simulink model "fullVehicleModel_17b"  (R2017b)
settings: Solver=VariableStepAuto  StartTime=0.0  StopTime=10.0  RelTol=1e-3
undefined symbols (not defined in the file): ambient_temp, bat, bat_r1, Batt, batt_initCharge, Batt_sensorLag_s, bvatt_AhRating, DiscIntNeverNeededParam, electronics_power, env, module_broad_area, module_small_area, module_top_area, mot, no_module, shifterPos, Ts, Ts_elec
libraries: Soft_ECUs x90, fl_lib x67, nesl_utility x29, Battery_lib x28, Gen_lib x13, simulink x10, aerolibconvert2 x7, SoftCAN_Interface x6, autolibshared x2, Additional_blocks_lib x1, elec_lib x1
(part 3 of 4)

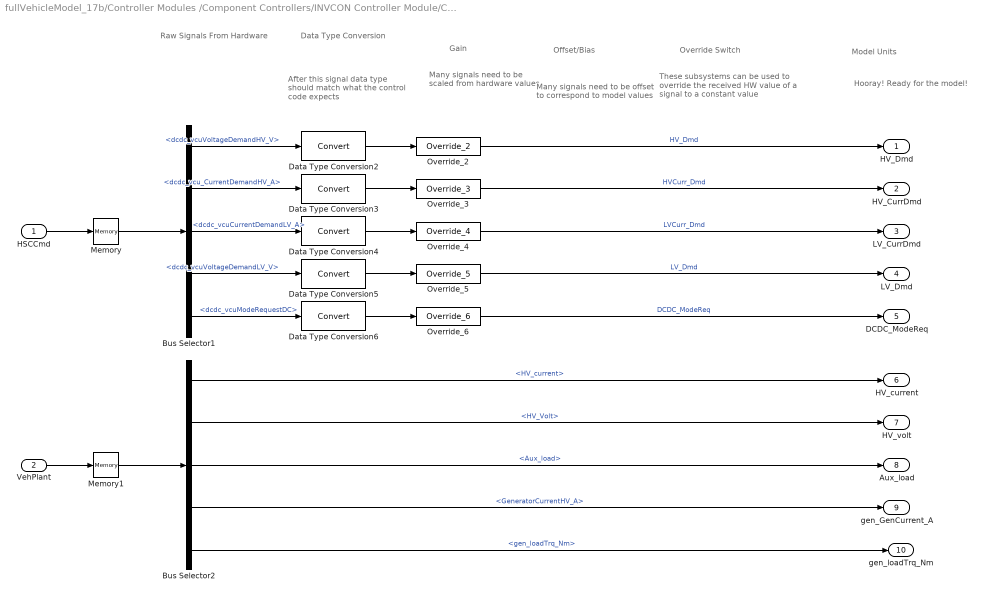
== system fullVehicleModel_17b/Controller Modules /Component Controllers/INVCON Controller Module/Controller Inputs/SiL Inputs ==
  note: Override Switch
  note: These subsystems can be used
      |  to override the received HW value
      | of a signal to a constant value
  note: Offset/Bias
  note: Many signals need
      | to be scaled from
      | hardware values
  note: Gain
  note: Raw Signals
      | From Hardware
  note: Model Units
  note: Hooray! Ready for
      | the model!
  note: After this signal data
      | type should match what
      | the control code expects
  note: Data Type
      | Conversion
  note: Many signals need
      | to be offset to correspond
      | to model values
  HSCCmd : Inport
  VehPlant : Inport  Port=2
  Bus Selector1 : BusSelector  OutputSignals=dcdc_vcuVoltageDemandHV_V,dcdc_vcu_CurrentDemandHV_A,dcdc_vcuCurrentDemandLV_A,dcdc_vcuVoltageDemandLV_V,dcdc_vcuModeRequestDC
  Bus Selector2 : BusSelector  OutputSignals=HV_current,HV_Volt,Aux_load,GeneratorCurrentHV_A,gen_loadTrq_Nm
  Data Type Conversion{2..6} (5 alike) : DataTypeConversion
  Memory : Memory
  Memory1 : Memory
  Override_2 : Gen_lib/INVCON_SoftECU2/SignalIn_Conversion_FIU/Override_2
  Override_3 : Gen_lib/INVCON_SoftECU2/SignalIn_Conversion_FIU/Override_3
  Override_4 : Gen_lib/INVCON_SoftECU2/SignalIn_Conversion_FIU/Override_4
  Override_5 : Gen_lib/INVCON_SoftECU2/SignalIn_Conversion_FIU/Override_5
  Override_6 : Gen_lib/INVCON_SoftECU2/SignalIn_Conversion_FIU/Override_6
  HV_Dmd : Outport
  HV_CurrDmd : Outport  Port=2
  LV_CurrDmd : Outport  Port=3
  LV_Dmd : Outport  Port=4
  DCDC_ModeReq : Outport  Port=5
  HV_current : Outport  Port=6
  HV_volt : Outport  Port=7
  Aux_load : Outport  Port=8
  gen_GenCurrent_A : Outport  Port=9
  gen_loadTrq_Nm : Outport  Port=10
  wires:
  Bus Selector1/4 -> Data Type Conversion5/1  "<dcdc_vcuVoltageDemandLV_V>"
  Override_6/1 -> DCDC_ModeReq/1  "DCDC_ModeReq"
  Override_3/1 -> HV_CurrDmd/1  "HVCurr_Dmd"
  Override_4/1 -> LV_CurrDmd/1  "LVCurr_Dmd"
  Bus Selector1/2 -> Data Type Conversion3/1  "<dcdc_vcu_CurrentDemandHV_A>"
  Bus Selector1/5 -> Data Type Conversion6/1  "<dcdc_vcuModeRequestDC>"
  Override_2/1 -> HV_Dmd/1  "HV_Dmd"
  Data Type Conversion5/1 -> Override_5/1
  Bus Selector1/3 -> Data Type Conversion4/1  "<dcdc_vcuCurrentDemandLV_A>"
  Data Type Conversion3/1 -> Override_3/1
  HSCCmd/1 -> Memory/1
  Data Type Conversion6/1 -> Override_6/1
  Bus Selector1/1 -> Data Type Conversion2/1  "<dcdc_vcuVoltageDemandHV_V>"
  Data Type Conversion2/1 -> Override_2/1
  Override_5/1 -> LV_Dmd/1  "LV_Dmd"
  Data Type Conversion4/1 -> Override_4/1
  Memory/1 -> Bus Selector1/1
  Bus Selector2/5 -> gen_loadTrq_Nm/1  "<gen_loadTrq_Nm>"
  Bus Selector2/2 -> HV_volt/1  "<HV_Volt>"
  Bus Selector2/1 -> HV_current/1  "<HV_current>"
  Bus Selector2/4 -> gen_GenCurrent_A/1  "<GeneratorCurrentHV_A>"
  Bus Selector2/3 -> Aux_load/1  "<Aux_load>"
  Memory1/1 -> Bus Selector2/1
  VehPlant/1 -> Memory1/1

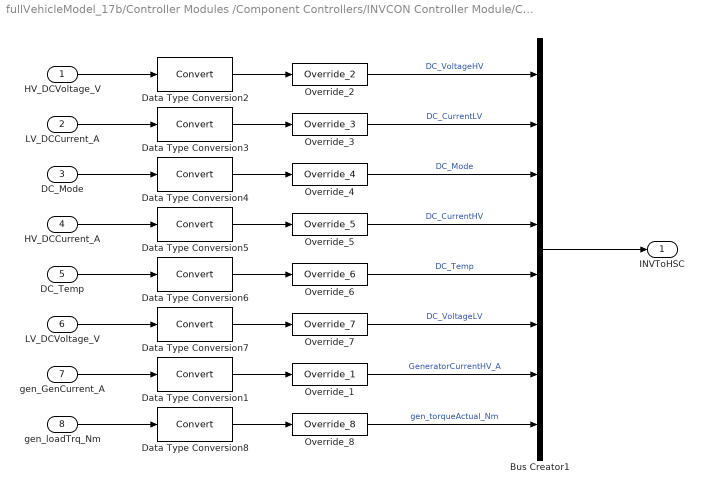
== system fullVehicleModel_17b/Controller Modules /Component Controllers/INVCON Controller Module/Controller Outputs/SiL Controller Outputs ==
  HV_DCVoltage_V : Inport
  LV_DCCurrent_A : Inport  Port=2
  DC_Mode : Inport  Port=3
  HV_DCCurrent_A : Inport  Port=4
  DC_Temp : Inport  Port=5
  LV_DCVoltage_V : Inport  Port=6
  gen_GenCurrent_A : Inport  Port=7
  gen_loadTrq_Nm : Inport  Port=8
  Bus Creator1 : BusCreator  Inputs=8
  Data Type Conversion{1..8} (8 alike) : DataTypeConversion
  Override_1 : Gen_lib/INVCON_SoftECU2/SignalOut_Conversion_FIU/Override_1
  Override_2 : Gen_lib/INVCON_SoftECU2/SignalOut_Conversion_FIU/Override_2
  Override_3 : Gen_lib/INVCON_SoftECU2/SignalOut_Conversion_FIU/Override_3
  Override_4 : Gen_lib/INVCON_SoftECU2/SignalOut_Conversion_FIU/Override_4
  Override_5 : Gen_lib/INVCON_SoftECU2/SignalOut_Conversion_FIU/Override_5
  Override_6 : Gen_lib/INVCON_SoftECU2/SignalOut_Conversion_FIU/Override_6
  Override_7 : Gen_lib/INVCON_SoftECU2/SignalOut_Conversion_FIU/Override_7
  Override_8 : Gen_lib/INVCON_SoftECU2/SignalOut_Conversion_FIU/Override_8
  INVToHSC : Outport
  wires:
  Data Type Conversion8/1 -> Override_8/1
  Data Type Conversion3/1 -> Override_3/1
  Override_8/1 -> Bus Creator1/8  "gen_torqueActual_Nm"
  Bus Creator1/1 -> INVToHSC/1
  Data Type Conversion4/1 -> Override_4/1
  Data Type Conversion2/1 -> Override_2/1
  Override_2/1 -> Bus Creator1/1  "DC_VoltageHV"
  Override_1/1 -> Bus Creator1/7  "GeneratorCurrentHV_A"
  Data Type Conversion5/1 -> Override_5/1
  Data Type Conversion6/1 -> Override_6/1
  Data Type Conversion7/1 -> Override_7/1
  Data Type Conversion1/1 -> Override_1/1
  Override_4/1 -> Bus Creator1/3  "DC_Mode"
  Override_7/1 -> Bus Creator1/6  "DC_VoltageLV"
  Override_3/1 -> Bus Creator1/2  "DC_CurrentLV"
  Override_6/1 -> Bus Creator1/5  "DC_Temp"
  Override_5/1 -> Bus Creator1/4  "DC_CurrentHV"
  HV_DCVoltage_V/1 -> Data Type Conversion2/1
  LV_DCCurrent_A/1 -> Data Type Conversion3/1
  DC_Mode/1 -> Data Type Conversion4/1
  HV_DCCurrent_A/1 -> Data Type Conversion5/1
  DC_Temp/1 -> Data Type Conversion6/1
  LV_DCVoltage_V/1 -> Data Type Conversion7/1
  gen_GenCurrent_A/1 -> Data Type Conversion1/1
  gen_loadTrq_Nm/1 -> Data Type Conversion8/1

== system fullVehicleModel_17b/Controller Modules /Component Controllers/INVCON Controller Module/INVCON Controller Module/Conditional Divide ==
  u1 : Inport
  u2 : Inport  Port=2
  u3 : Inport  Port=3
  Constant1 : Constant  Value=eps
  Constant3 : Constant  Value=0
  Divide : Product  Inputs=/*
  Logical Operator : Logic  Operator=NOT  AllPortsSameDT=off  OutDataTypeStr=boolean
  Relational Operator : RelationalOperator  Operator===  OutDataTypeStr=boolean  RndMeth=Nearest
  Switch : Switch  Criteria=u2 ~= 0
  Switch1 : Switch  Criteria=u2 ~= 0
  Out1 : Outport
  wires:
  Constant3/1 -> Relational Operator/2
  Divide/1 -> Switch1/1
  u2/1 -> Relational Operator/1, Switch/3
  u1/1 -> Divide/2
  Relational Operator/1 -> Switch/2, Logical Operator/1
  u3/1 -> Switch1/3
  Constant1/1 -> Switch/1
  Switch1/1 -> Out1/1
  Logical Operator/1 -> Switch1/2
  Switch/1 -> Divide/1

== system fullVehicleModel_17b/Controller Modules /Component Controllers/Left Motor Control Module/Controller/Fault Daignosis ==
  current : Inport
  voltage : Inport  Port=2
  temp : Inport  Port=3
  Bus Creator : BusCreator  Inputs=5
  Device Temp to High : Subsystem
  Motor Temp to High : Subsystem
  No Power Supply Voltage : Subsystem
  Over Current : Subsystem
  Over Voltage : Subsystem
  Fault Message : Outport
  wires:
  Bus Creator/1 -> Fault Message/1
  Over Current/1(Out1) -> Bus Creator/5  "mot_fault_iPeak"
  Over Voltage/1(Out1) -> Bus Creator/2  "mot_fault_overVoltage"
  Device Temp to High/1(Out1) -> Bus Creator/4  "mot_fault_deviceTemp"
  Motor Temp to High/1(Out1) -> Bus Creator/3  "mot_fault_mtrTemp"
  No Power Supply Voltage/1(Out1) -> Bus Creator/1  "mot_fault_pwrVoltage"
  temp/1 -> Motor Temp to High/1(Mot_temp), Device Temp to High/1(Device Temp)
  current/1 -> Over Current/1(Motor Current)
  voltage/1 -> Over Voltage/1(Device Voltage), No Power Supply Voltage/1(mot_voltage)

== system fullVehicleModel_17b/Controller Modules /Component Controllers/Left Motor Control Module/Controller/Motor CMD ==
  note: This subsystem is used to override the model value of a signal to a constant value
  note: Override Switch Subsystem
  trq_cmd : Inport
  mot_mode : Inport  Port=2
  Multiport Switch : MultiPortSwitch  DataPortOrder=Zero-based contiguous  Inputs=2  zeroidx=on
  Override Value : Constant  Value=0
  Out1 : Outport
  wires:
  mot_mode/1 -> Multiport Switch/1
  Override Value/1 -> Multiport Switch/2
  trq_cmd/1 -> Multiport Switch/3
  Multiport Switch/1 -> Out1/1

== system fullVehicleModel_17b/Controller Modules /Component Controllers/Left Motor Control Module/Controller/Subsystem ==
  voltage : Inport
  speed : Inport  Port=2
  current : Inport  Port=3
  mode : Inport  Port=4
  Out1 : Outport

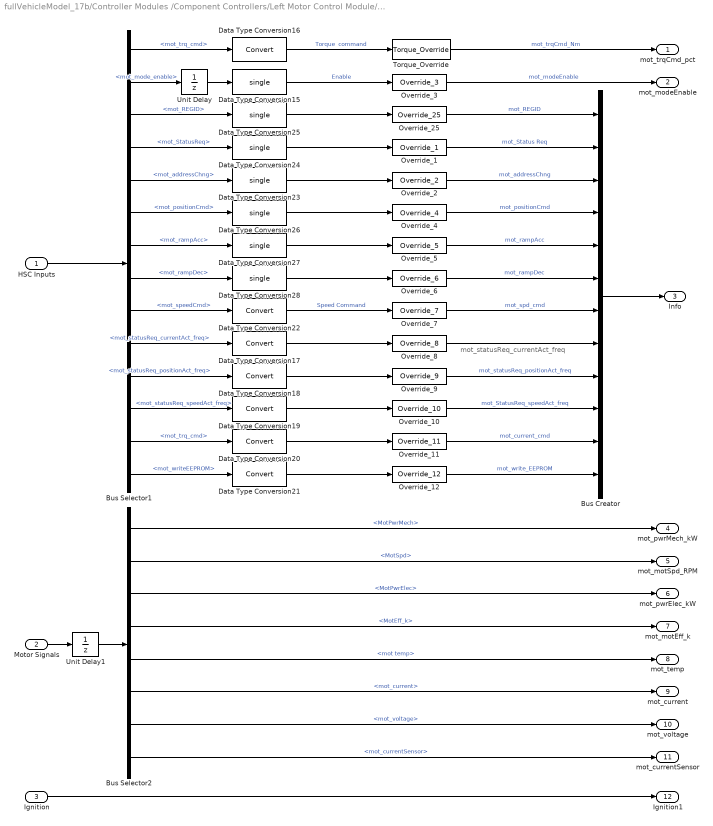
== system fullVehicleModel_17b/Controller Modules /Component Controllers/Left Motor Control Module/Controller Inputs/SiL Inputs ==
  note: mot_statusReq_currentAct_freq
  HSC Inputs : Inport
  Motor Signals : Inport  Port=2
  Ignition : Inport  Port=3
  Bus Creator : BusCreator  Inputs=12
  Bus Selector1 : BusSelector  OutputSignals=mot_trq_cmd,mot_mode_enable,mot_REGID,mot_StatusReq,mot_addressChng,mot_positionCmd,mot_rampAcc,mot_rampDec,mot_speedCmd,mot_statusReq_currentAct_freq,mot_statusReq_positionAct_freq,mot_statusReq_speedAct_freq,mot_trq_cmd,mot_writeEEPROM
  Bus Selector2 : BusSelector  OutputSignals=MotPwrMech,MotSpd,MotPwrElec,MotEff_k,mot temp,mot_current,mot_voltage,mot_currentSensor
  Data Type Conversion{15,23..28} (7 alike) : DataTypeConversion  OutDataTypeStr=single
  Data Type Conversion{16..22} (7 alike) : DataTypeConversion
  Override_1 : Soft_ECUs/softECU_Motor/Conversion/Override_1
  Override_10 : Soft_ECUs/softECU_Motor/Conversion/Override_10
  Override_11 : Soft_ECUs/softECU_Motor/Conversion/Override_11
  Override_12 : Soft_ECUs/softECU_Motor/Conversion/Override_12
  Override_2 : Soft_ECUs/softECU_Motor/Conversion/Override_2
  Override_25 : Soft_ECUs/softECU_Motor/Conversion/Override_25
  Override_3 : Soft_ECUs/softECU_Motor/Conversion/Override_3
  Override_4 : Soft_ECUs/softECU_Motor/Conversion/Override_4
  Override_5 : Soft_ECUs/softECU_Motor/Conversion/Override_5
  Override_6 : Soft_ECUs/softECU_Motor/Conversion/Override_6
  Override_7 : Soft_ECUs/softECU_Motor/Conversion/Override_7
  Override_8 : Soft_ECUs/softECU_Motor/Conversion/Override_8
  Override_9 : Soft_ECUs/softECU_Motor/Conversion/Override_9
  Torque_Override : Soft_ECUs/softECU_Motor/Conversion/Torque_Override
  Unit Delay : UnitDelay  SampleTime=-1
  Unit Delay1 : UnitDelay  SampleTime=-1
  mot_trqCmd_pct : Outport
  mot_modeEnable : Outport  Port=2
  Info : Outport  Port=3
  mot_pwrMech_kW : Outport  Port=4
  mot_motSpd_RPM : Outport  Port=5
  mot_pwrElec_kW : Outport  Port=6
  mot_motEff_k : Outport  Port=7
  mot_temp : Outport  Port=8
  mot_current : Outport  Port=9
  mot_voltage : Outport  Port=10
  mot_currentSensor : Outport  Port=11
  Ignition1 : Outport  Port=12
  wires:
  Override_12/1 -> Bus Creator/12  "mot_write_EEPROM"
  Data Type Conversion24/1 -> Override_1/1
  Bus Selector1/14 -> Data Type Conversion21/1  "<mot_writeEEPROM>"
  Override_6/1 -> Bus Creator/6  "mot_rampDec"
  Bus Selector1/13 -> Data Type Conversion20/1  "<mot_trq_cmd>"
  Override_1/1 -> Bus Creator/2  "mot_Status Req"
  Bus Selector1/7 -> Data Type Conversion27/1  "<mot_rampAcc>"
  Data Type Conversion22/1 -> Override_7/1  "Speed Command"
  Bus Selector1/12 -> Data Type Conversion19/1  "<mot_statusReq_speedAct_freq>"
  Data Type Conversion17/1 -> Override_8/1
  Data Type Conversion18/1 -> Override_9/1
  Override_9/1 -> Bus Creator/9  "mot_statusReq_positionAct_freq"
  Bus Selector1/11 -> Data Type Conversion18/1  "<mot_statusReq_positionAct_freq>"
  Override_10/1 -> Bus Creator/10  "mot_StatusReq_speedAct_freq"
  Override_4/1 -> Bus Creator/4  "mot_positionCmd"
  Data Type Conversion27/1 -> Override_5/1
  Override_8/1 -> Bus Creator/8
  Data Type Conversion23/1 -> Override_2/1
  Override_11/1 -> Bus Creator/11  "mot_current_cmd"
  Data Type Conversion25/1 -> Override_25/1
  Bus Selector1/6 -> Data Type Conversion26/1  "<mot_positionCmd>"
  Data Type Conversion28/1 -> Override_6/1
  Override_7/1 -> Bus Creator/7  "mot_spd_cmd"
  Bus Selector1/5 -> Data Type Conversion23/1  "<mot_addressChng>"
  Data Type Conversion26/1 -> Override_4/1
  Bus Selector1/8 -> Data Type Conversion28/1  "<mot_rampDec>"
  Bus Selector1/1 -> Data Type Conversion16/1  "<mot_trq_cmd>"
  Data Type Conversion19/1 -> Override_10/1
  Bus Selector1/3 -> Data Type Conversion25/1  "<mot_REGID>"
  Override_25/1 -> Bus Creator/1  "mot_REGID"
  Bus Selector1/4 -> Data Type Conversion24/1  "<mot_StatusReq>"
  Data Type Conversion21/1 -> Override_12/1
  Override_2/1 -> Bus Creator/3  "mot_addressChng"
  Data Type Conversion16/1 -> Torque_Override/1  "Torque  command"
  Override_5/1 -> Bus Creator/5  "mot_rampAcc"
  Bus Selector1/2 -> Unit Delay/1  "<mot_mode_enable>"
  Bus Selector1/9 -> Data Type Conversion22/1  "<mot_speedCmd>"
  Unit Delay/1 -> Data Type Conversion15/1
  HSC Inputs/1 -> Bus Selector1/1
  Data Type Conversion15/1 -> Override_3/1  "Enable"
  Bus Selector1/10 -> Data Type Conversion17/1  "<mot_statusReq_currentAct_freq>"
  Data Type Conversion20/1 -> Override_11/1
  Bus Selector2/5 -> mot_temp/1  "<mot temp>"
  Bus Selector2/6 -> mot_current/1  "<mot_current>"
  Bus Selector2/4 -> mot_motEff_k/1  "<MotEff_k>"
  Bus Selector2/3 -> mot_pwrElec_kW/1  "<MotPwrElec>"
  Bus Selector2/2 -> mot_motSpd_RPM/1  "<MotSpd>"
  Bus Selector2/1 -> mot_pwrMech_kW/1  "<MotPwrMech>"
  Motor Signals/1 -> Unit Delay1/1
  Bus Selector2/7 -> mot_voltage/1  "<mot_voltage>"
  Bus Selector2/8 -> mot_currentSensor/1  "<mot_currentSensor>"
  Bus Creator/1 -> Info/1
  Override_3/1 -> mot_modeEnable/1  "mot_modeEnable"
  Torque_Override/1 -> mot_trqCmd_pct/1  "mot_trqCmd_Nm"
  Ignition/1 -> Ignition1/1
  Unit Delay1/1 -> Bus Selector2/1

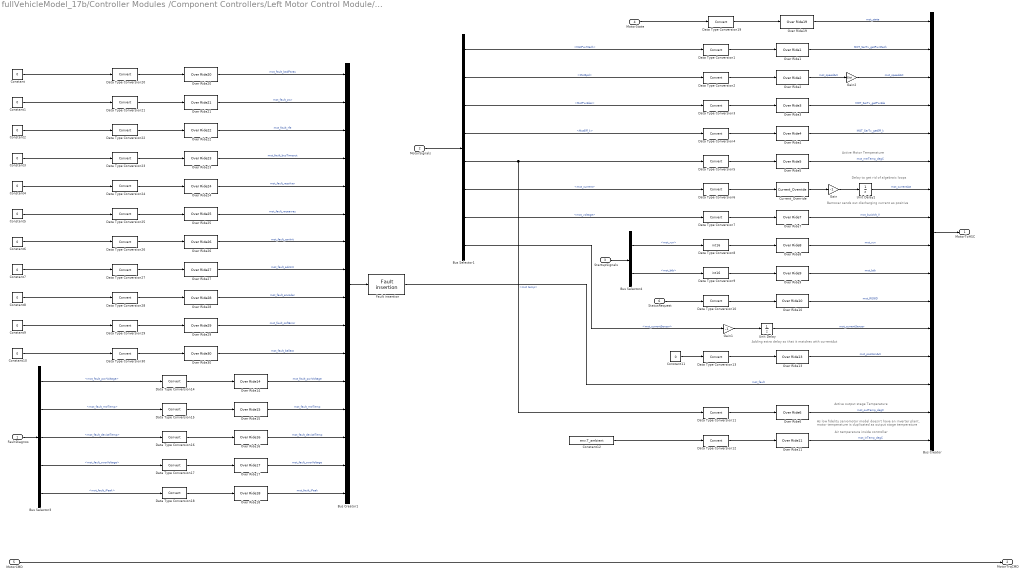
== system fullVehicleModel_17b/Controller Modules /Component Controllers/Left Motor Control Module/Controller Outputs/SiL Controller Outputs ==
  note: Active Motor Temperature
  note: Adding extra delay so that it matches with currentAct
  note: As low fidelity servomotor model doesn't have an inverter plant,
      | motor temperature is duplicated as output stage temperature
  note: Air temperature inside controller
  note: Delay to get rid of algebraic loops
  note: Active output stage Temperature
  note: Bamocar sends out discharging current as positive
  FaultDiagnos : Inport
  MotorSignals : Inport  Port=2
  StartupSignals : Inport  Port=3
  MotorState : Inport  Port=4
  MotorCMD : Inport  Port=5
  StatusRequest : Inport  Port=6
  Bus Creator : BusCreator  Inputs=16
  Bus Creator1 : BusCreator  Inputs=16
  Bus Selector1 : BusSelector  OutputSignals=MotPwrMech,MotSpd,MotPwrElec,MotEff_k,mot temp,mot_current,mot_voltage,mot_currentSensor
  Bus Selector3 : BusSelector  OutputSignals=mot_fault_pwrVoltage,mot_fault_mtrTemp,mot_fault_deviceTemp,mot_fault_overVoltage,mot_fault_iPeak
  Bus Selector4 : BusSelector  OutputSignals=mot_run,mot_btb
  Constant{,1..11} (12 alike) : Constant  Value=0
  Constant12 : Constant  Value=env.T_ambient
  Current_Override : Soft_ECUs/softECU_Motor/conversion 2/Current_Override
  Data Type Conversion{1..7,10..30} (28 alike) : DataTypeConversion
  Data Type Conversion8 : DataTypeConversion  OutDataTypeStr=int16
  Data Type Conversion9 : DataTypeConversion  OutDataTypeStr=int16
  Fault insertion : Soft_ECUs/softECU_Motor/conversion 2/Fault insertion
  Gain : Gain  Gain=-1
  Gain1 : Gain  Gain=-1
  Gain2 : Gain  Gain=30/pi
  Over Ride1 : Soft_ECUs/softECU_Motor/conversion 2/Over Ride1
  Over Ride10 : Soft_ECUs/softECU_Motor/conversion 2/Over Ride10
  Over Ride11 : Soft_ECUs/softECU_Motor/conversion 2/Over Ride11
  Over Ride13 : Soft_ECUs/softECU_Motor/conversion 2/Over Ride13
  Over Ride14 : Soft_ECUs/softECU_Motor/conversion 2/Over Ride14
  Over Ride15 : Soft_ECUs/softECU_Motor/conversion 2/Over Ride15
  Over Ride16 : Soft_ECUs/softECU_Motor/conversion 2/Over Ride16
  Over Ride17 : Soft_ECUs/softECU_Motor/conversion 2/Over Ride17
  Over Ride18 : Soft_ECUs/softECU_Motor/conversion 2/Over Ride18
  Over Ride19 : Soft_ECUs/softECU_Motor/conversion 2/Over Ride19
  Over Ride2 : Soft_ECUs/softECU_Motor/conversion 2/Over Ride2
  Over Ride20 : Soft_ECUs/softECU_Motor/conversion 2/Over Ride20
  Over Ride21 : Soft_ECUs/softECU_Motor/conversion 2/Over Ride21
  Over Ride22 : Soft_ECUs/softECU_Motor/conversion 2/Over Ride22
  Over Ride23 : Soft_ECUs/softECU_Motor/conversion 2/Over Ride23
  Over Ride24 : Soft_ECUs/softECU_Motor/conversion 2/Over Ride24
  Over Ride25 : Soft_ECUs/softECU_Motor/conversion 2/Over Ride25
  Over Ride26 : Soft_ECUs/softECU_Motor/conversion 2/Over Ride26
  Over Ride27 : Soft_ECUs/softECU_Motor/conversion 2/Over Ride27
  Over Ride28 : Soft_ECUs/softECU_Motor/conversion 2/Over Ride28
  Over Ride29 : Soft_ECUs/softECU_Motor/conversion 2/Over Ride29
  Over Ride3 : Soft_ECUs/softECU_Motor/conversion 2/Over Ride3
  Over Ride30 : Soft_ECUs/softECU_Motor/conversion 2/Over Ride30
  Over Ride4 : Soft_ECUs/softECU_Motor/conversion 2/Over Ride4
  Over Ride5 : Soft_ECUs/softECU_Motor/conversion 2/Over Ride5
  Over Ride6 : Soft_ECUs/softECU_Motor/conversion 2/Over Ride6
  Over Ride7 : Soft_ECUs/softECU_Motor/conversion 2/Over Ride7
  Over Ride8 : Soft_ECUs/softECU_Motor/conversion 2/Over Ride8
  Over Ride9 : Soft_ECUs/softECU_Motor/conversion 2/Over Ride9
  Unit Delay : UnitDelay  SampleTime=-1
  Unit Delay1 : UnitDelay  SampleTime=-1
  MotorToHSC : Outport
  MotorTrqCMD : Outport  Port=2
  wires:
  Data Type Conversion13/1 -> Over Ride13/1
  Over Ride10/1 -> Bus Creator/11  "mot_REGID"
  StatusRequest/1 -> Data Type Conversion10/1
  MotorState/1 -> Data Type Conversion19/1
  Over Ride8/1 -> Bus Creator/9  "mot_run"
  Constant10/1 -> Data Type Conversion30/1
  Bus Selector1/3 -> Data Type Conversion3/1  "<MotPwrElec>"
  Over Ride9/1 -> Bus Creator/10  "mot_btb"
  Data Type Conversion9/1 -> Over Ride9/1
  Data Type Conversion21/1 -> Over Ride21/1
  StartupSignals/1 -> Bus Selector4/1
  MotorSignals/1 -> Bus Selector1/1
  Bus Selector4/2 -> Data Type Conversion9/1  "<mot_btb>"
  Bus Selector1/2 -> Data Type Conversion2/1  "<MotSpd>"
  Data Type Conversion5/1 -> Over Ride5/1
  Data Type Conversion28/1 -> Over Ride28/1
  Bus Selector4/1 -> Data Type Conversion8/1  "<mot_run>"
  Bus Selector1/7 -> Data Type Conversion7/1  "<mot_voltage>"
  Current_Override/1 -> Gain/1
  Bus Selector3/1 -> Data Type Conversion14/1  "<mot_fault_pwrVoltage>"
  Over Ride18/1 -> Bus Creator1/16  "mot_fault_iPeak"
  Over Ride16/1 -> Bus Creator1/14  "mot_fault_deviceTemp"
  Over Ride14/1 -> Bus Creator1/12  "mot_fault_pwrVoltage"
  Data Type Conversion1/1 -> Over Ride1/1
  Constant9/1 -> Data Type Conversion29/1
  Constant/1 -> Data Type Conversion20/1
  Data Type Conversion10/1 -> Over Ride10/1
  Data Type Conversion23/1 -> Over Ride23/1
  Data Type Conversion3/1 -> Over Ride3/1
  Data Type Conversion8/1 -> Over Ride8/1
  Data Type Conversion4/1 -> Over Ride4/1
  Bus Selector1/1 -> Data Type Conversion1/1  "<MotPwrMech>"
  Bus Selector1/5 -> Data Type Conversion5/1, Data Type Conversion11/1  "<mot temp>"
  Over Ride3/1 -> Bus Creator/4  "MOT_SerTx_getPwrEle"
  Over Ride5/1 -> Bus Creator/6  "mot_mtrTemp_degC"
  FaultDiagnos/1 -> Bus Selector3/1
  Bus Selector3/2 -> Data Type Conversion15/1  "<mot_fault_mtrTemp>"
  Bus Selector3/3 -> Data Type Conversion16/1  "<mot_fault_deviceTemp>"
  Data Type Conversion20/1 -> Over Ride20/1
  Constant11/1 -> Data Type Conversion13/1
  Data Type Conversion24/1 -> Over Ride24/1
  Over Ride7/1 -> Bus Creator/8  "mot_busVolt_V"
  Data Type Conversion19/1 -> Over Ride19/1
  Over Ride13/1 -> Bus Creator/13  "mot_positionAct"
  Over Ride19/1 -> Bus Creator/1  "mot_state"
  Bus Creator1/1 -> Fault insertion/1
  Data Type Conversion22/1 -> Over Ride22/1
  Gain2/1 -> Bus Creator/3  "mot_speedAct"
  Over Ride21/1 -> Bus Creator1/2  "mot_fault_pwr"
  Over Ride15/1 -> Bus Creator1/13  "mot_fault_mtrTemp"
  Data Type Conversion2/1 -> Over Ride2/1
  Data Type Conversion7/1 -> Over Ride7/1
  Over Ride20/1 -> Bus Creator1/1  "mot_fault_badParas"
  Data Type Conversion30/1 -> Over Ride30/1
  Bus Creator/1 -> MotorToHSC/1
  Over Ride6/1 -> Bus Creator/15  "mot_outTemp_degC"
  Over Ride25/1 -> Bus Creator1/6  "mot_fault_raceaway"
  Bus Selector3/4 -> Data Type Conversion17/1  "<mot_fault_overVoltage>"
  Over Ride1/1 -> Bus Creator/2  "MOT_SerTx_getPwrMech"
  Over Ride30/1 -> Bus Creator1/11  "mot_fault_ballast"
  Constant7/1 -> Data Type Conversion27/1
  Unit Delay/1 -> Bus Creator/12  "mot_currentSensor"
  Data Type Conversion18/1 -> Over Ride18/1
  Bus Selector1/8 -> Gain1/1  "<mot_currentSensor>"
  Gain1/1 -> Unit Delay/1
  Data Type Conversion11/1 -> Over Ride6/1
  Data Type Conversion12/1 -> Over Ride11/1
  Constant8/1 -> Data Type Conversion28/1
  Data Type Conversion6/1 -> Current_Override/1
  Data Type Conversion16/1 -> Over Ride16/1
  Over Ride22/1 -> Bus Creator1/3  "mot_fault_rfe"
  Constant1/1 -> Data Type Conversion21/1
  Data Type Conversion29/1 -> Over Ride29/1
  Fault insertion/1 -> Bus Creator/14  "mot_fault"
  Constant3/1 -> Data Type Conversion23/1
  Over Ride26/1 -> Bus Creator1/7  "mot_fault_canInit"
  Over Ride4/1 -> Bus Creator/5  "MOT_SerTx_getEff_k"
  Constant2/1 -> Data Type Conversion22/1
  Data Type Conversion14/1 -> Over Ride14/1
  Bus Selector1/4 -> Data Type Conversion4/1  "<MotEff_k>"
  Over Ride11/1 -> Bus Creator/16  "mot_inTemp_degC"
  Data Type Conversion25/1 -> Over Ride25/1
  Constant5/1 -> Data Type Conversion25/1
  Bus Selector1/6 -> Data Type Conversion6/1  "<mot_current>"
  Data Type Conversion26/1 -> Over Ride26/1
  Data Type Conversion27/1 -> Over Ride27/1
  Over Ride24/1 -> Bus Creator1/5  "mot_fault_resolver"
  Gain/1 -> Unit Delay1/1
  Over Ride2/1 -> Gain2/1  "mot_speedAct"
  Unit Delay1/1 -> Bus Creator/7  "mot_currentAct"
  Bus Selector3/5 -> Data Type Conversion18/1  "<mot_fault_iPeak>"
  Over Ride28/1 -> Bus Creator1/9  "mot_fault_encoder"
  Data Type Conversion17/1 -> Over Ride17/1
  Constant12/1 -> Data Type Conversion12/1
  Over Ride27/1 -> Bus Creator1/8  "mot_fault_adcInit"
  Over Ride17/1 -> Bus Creator1/15  "mot_fault_overVoltage"
  Over Ride23/1 -> Bus Creator1/4  "mot_fault_busTimeout"
  Data Type Conversion15/1 -> Over Ride15/1
  Constant6/1 -> Data Type Conversion26/1
  Constant4/1 -> Data Type Conversion24/1
  Over Ride29/1 -> Bus Creator1/10  "mot_fault_softError"
  MotorCMD/1 -> MotorTrqCMD/1

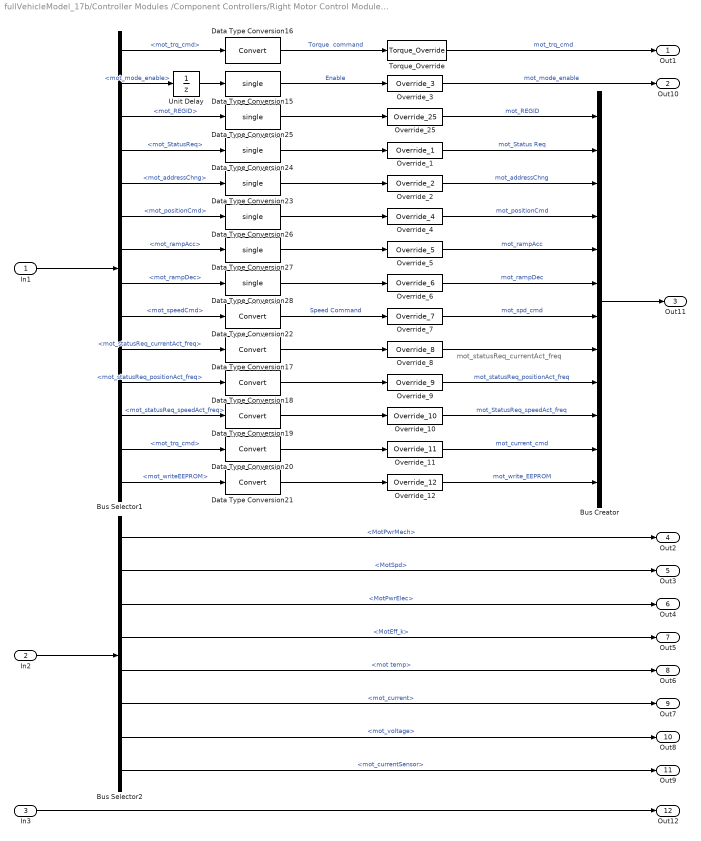
== system fullVehicleModel_17b/Controller Modules /Component Controllers/Right Motor Control Module/Controller Inputs/SiL Inputs ==
  note: mot_statusReq_currentAct_freq
  In1 : Inport
  In2 : Inport  Port=2
  In3 : Inport  Port=3
  Bus Creator : BusCreator  Inputs=12
  Bus Selector1 : BusSelector  OutputSignals=mot_trq_cmd,mot_mode_enable,mot_REGID,mot_StatusReq,mot_addressChng,mot_positionCmd,mot_rampAcc,mot_rampDec,mot_speedCmd,mot_statusReq_currentAct_freq,mot_statusReq_positionAct_freq,mot_statusReq_speedAct_freq,mot_trq_cmd,mot_writeEEPROM
  Bus Selector2 : BusSelector  OutputSignals=MotPwrMech,MotSpd,MotPwrElec,MotEff_k,mot temp,mot_current,mot_voltage,mot_currentSensor
  Data Type Conversion{15,23..28} (7 alike) : DataTypeConversion  OutDataTypeStr=single
  Data Type Conversion{16..22} (7 alike) : DataTypeConversion
  Override_1 : Soft_ECUs/softECU_Motor/Conversion/Override_1
  Override_10 : Soft_ECUs/softECU_Motor/Conversion/Override_10
  Override_11 : Soft_ECUs/softECU_Motor/Conversion/Override_11
  Override_12 : Soft_ECUs/softECU_Motor/Conversion/Override_12
  Override_2 : Soft_ECUs/softECU_Motor/Conversion/Override_2
  Override_25 : Soft_ECUs/softECU_Motor/Conversion/Override_25
  Override_3 : Soft_ECUs/softECU_Motor/Conversion/Override_3
  Override_4 : Soft_ECUs/softECU_Motor/Conversion/Override_4
  Override_5 : Soft_ECUs/softECU_Motor/Conversion/Override_5
  Override_6 : Soft_ECUs/softECU_Motor/Conversion/Override_6
  Override_7 : Soft_ECUs/softECU_Motor/Conversion/Override_7
  Override_8 : Soft_ECUs/softECU_Motor/Conversion/Override_8
  Override_9 : Soft_ECUs/softECU_Motor/Conversion/Override_9
  Torque_Override : Soft_ECUs/softECU_Motor/Conversion/Torque_Override
  Unit Delay : UnitDelay  SampleTime=-1
  Out1 : Outport
  Out10 : Outport  Port=2
  Out11 : Outport  Port=3
  Out2 : Outport  Port=4
  Out3 : Outport  Port=5
  Out4 : Outport  Port=6
  Out5 : Outport  Port=7
  Out6 : Outport  Port=8
  Out7 : Outport  Port=9
  Out8 : Outport  Port=10
  Out9 : Outport  Port=11
  Out12 : Outport  Port=12
  wires:
  Override_12/1 -> Bus Creator/12  "mot_write_EEPROM"
  Data Type Conversion24/1 -> Override_1/1
  Bus Selector1/14 -> Data Type Conversion21/1  "<mot_writeEEPROM>"
  Override_6/1 -> Bus Creator/6  "mot_rampDec"
  Bus Selector1/13 -> Data Type Conversion20/1  "<mot_trq_cmd>"
  Override_1/1 -> Bus Creator/2  "mot_Status Req"
  Bus Selector1/7 -> Data Type Conversion27/1  "<mot_rampAcc>"
  Data Type Conversion22/1 -> Override_7/1  "Speed Command"
  Bus Selector1/12 -> Data Type Conversion19/1  "<mot_statusReq_speedAct_freq>"
  Data Type Conversion17/1 -> Override_8/1
  Data Type Conversion18/1 -> Override_9/1
  Override_9/1 -> Bus Creator/9  "mot_statusReq_positionAct_freq"
  Bus Selector1/11 -> Data Type Conversion18/1  "<mot_statusReq_positionAct_freq>"
  Override_10/1 -> Bus Creator/10  "mot_StatusReq_speedAct_freq"
  Override_4/1 -> Bus Creator/4  "mot_positionCmd"
  Data Type Conversion27/1 -> Override_5/1
  Override_8/1 -> Bus Creator/8
  Data Type Conversion23/1 -> Override_2/1
  Override_11/1 -> Bus Creator/11  "mot_current_cmd"
  Data Type Conversion25/1 -> Override_25/1
  Bus Selector1/6 -> Data Type Conversion26/1  "<mot_positionCmd>"
  Data Type Conversion28/1 -> Override_6/1
  Override_7/1 -> Bus Creator/7  "mot_spd_cmd"
  Bus Selector1/5 -> Data Type Conversion23/1  "<mot_addressChng>"
  Data Type Conversion26/1 -> Override_4/1
  Bus Selector1/8 -> Data Type Conversion28/1  "<mot_rampDec>"
  Bus Selector1/1 -> Data Type Conversion16/1  "<mot_trq_cmd>"
  Data Type Conversion19/1 -> Override_10/1
  Bus Selector1/3 -> Data Type Conversion25/1  "<mot_REGID>"
  Override_25/1 -> Bus Creator/1  "mot_REGID"
  Bus Selector1/4 -> Data Type Conversion24/1  "<mot_StatusReq>"
  Data Type Conversion21/1 -> Override_12/1
  Override_2/1 -> Bus Creator/3  "mot_addressChng"
  Data Type Conversion16/1 -> Torque_Override/1  "Torque  command"
  Override_5/1 -> Bus Creator/5  "mot_rampAcc"
  Bus Selector1/2 -> Unit Delay/1  "<mot_mode_enable>"
  Bus Selector1/9 -> Data Type Conversion22/1  "<mot_speedCmd>"
  Unit Delay/1 -> Data Type Conversion15/1
  In1/1 -> Bus Selector1/1
  Data Type Conversion15/1 -> Override_3/1  "Enable"
  Bus Selector1/10 -> Data Type Conversion17/1  "<mot_statusReq_currentAct_freq>"
  Data Type Conversion20/1 -> Override_11/1
  Bus Selector2/5 -> Out6/1  "<mot temp>"
  Bus Selector2/6 -> Out7/1  "<mot_current>"
  Bus Selector2/4 -> Out5/1  "<MotEff_k>"
  Bus Selector2/3 -> Out4/1  "<MotPwrElec>"
  Bus Selector2/2 -> Out3/1  "<MotSpd>"
  Bus Selector2/1 -> Out2/1  "<MotPwrMech>"
  In2/1 -> Bus Selector2/1
  Bus Selector2/7 -> Out8/1  "<mot_voltage>"
  Bus Selector2/8 -> Out9/1  "<mot_currentSensor>"
  Bus Creator/1 -> Out11/1
  Override_3/1 -> Out10/1  "mot_mode_enable"
  Torque_Override/1 -> Out1/1  "mot_trq_cmd"
  In3/1 -> Out12/1

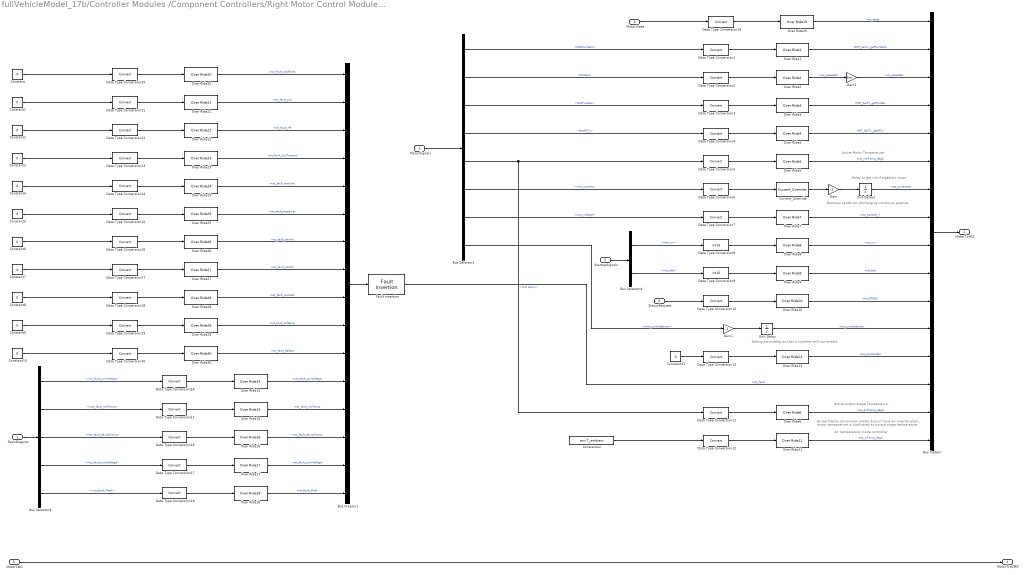
== system fullVehicleModel_17b/Controller Modules /Component Controllers/Right Motor Control Module/Controller Outputs/SiL Controller Outputs ==
  note: Active Motor Temperature
  note: Adding extra delay so that it matches with currentAct
  note: As low fidelity servomotor model doesn't have an inverter plant,
      | motor temperature is duplicated as output stage temperature
  note: Air temperature inside controller
  note: Delay to get rid of algebraic loops
  note: Active output stage Temperature
  note: Bamocar sends out discharging current as positive
  FaultDiagnos : Inport
  MotorSignals : Inport  Port=2
  StartupSignals : Inport  Port=3
  MotorState : Inport  Port=4
  MotorCMD : Inport  Port=5
  StatusRequest : Inport  Port=6
  Bus Creator : BusCreator  Inputs=16
  Bus Creator1 : BusCreator  Inputs=16
  Bus Selector1 : BusSelector  OutputSignals=MotPwrMech,MotSpd,MotPwrElec,MotEff_k,mot temp,mot_current,mot_voltage,mot_currentSensor
  Bus Selector3 : BusSelector  OutputSignals=mot_fault_pwrVoltage,mot_fault_mtrTemp,mot_fault_deviceTemp,mot_fault_overVoltage,mot_fault_iPeak
  Bus Selector4 : BusSelector  OutputSignals=mot_run,mot_btb
  Constant{,1..11} (12 alike) : Constant  Value=0
  Constant12 : Constant  Value=env.T_ambient
  Current_Override : Soft_ECUs/softECU_Motor/conversion 2/Current_Override
  Data Type Conversion{1..7,10..30} (28 alike) : DataTypeConversion
  Data Type Conversion8 : DataTypeConversion  OutDataTypeStr=int16
  Data Type Conversion9 : DataTypeConversion  OutDataTypeStr=int16
  Fault insertion : Soft_ECUs/softECU_Motor/conversion 2/Fault insertion
  Gain : Gain  Gain=-1
  Gain1 : Gain  Gain=-1
  Gain2 : Gain  Gain=30/pi
  Over Ride1 : Soft_ECUs/softECU_Motor/conversion 2/Over Ride1
  Over Ride10 : Soft_ECUs/softECU_Motor/conversion 2/Over Ride10
  Over Ride11 : Soft_ECUs/softECU_Motor/conversion 2/Over Ride11
  Over Ride13 : Soft_ECUs/softECU_Motor/conversion 2/Over Ride13
  Over Ride14 : Soft_ECUs/softECU_Motor/conversion 2/Over Ride14
  Over Ride15 : Soft_ECUs/softECU_Motor/conversion 2/Over Ride15
  Over Ride16 : Soft_ECUs/softECU_Motor/conversion 2/Over Ride16
  Over Ride17 : Soft_ECUs/softECU_Motor/conversion 2/Over Ride17
  Over Ride18 : Soft_ECUs/softECU_Motor/conversion 2/Over Ride18
  Over Ride19 : Soft_ECUs/softECU_Motor/conversion 2/Over Ride19
  Over Ride2 : Soft_ECUs/softECU_Motor/conversion 2/Over Ride2
  Over Ride20 : Soft_ECUs/softECU_Motor/conversion 2/Over Ride20
  Over Ride21 : Soft_ECUs/softECU_Motor/conversion 2/Over Ride21
  Over Ride22 : Soft_ECUs/softECU_Motor/conversion 2/Over Ride22
  Over Ride23 : Soft_ECUs/softECU_Motor/conversion 2/Over Ride23
  Over Ride24 : Soft_ECUs/softECU_Motor/conversion 2/Over Ride24
  Over Ride25 : Soft_ECUs/softECU_Motor/conversion 2/Over Ride25
  Over Ride26 : Soft_ECUs/softECU_Motor/conversion 2/Over Ride26
  Over Ride27 : Soft_ECUs/softECU_Motor/conversion 2/Over Ride27
  Over Ride28 : Soft_ECUs/softECU_Motor/conversion 2/Over Ride28
  Over Ride29 : Soft_ECUs/softECU_Motor/conversion 2/Over Ride29
  Over Ride3 : Soft_ECUs/softECU_Motor/conversion 2/Over Ride3
  Over Ride30 : Soft_ECUs/softECU_Motor/conversion 2/Over Ride30
  Over Ride4 : Soft_ECUs/softECU_Motor/conversion 2/Over Ride4
  Over Ride5 : Soft_ECUs/softECU_Motor/conversion 2/Over Ride5
  Over Ride6 : Soft_ECUs/softECU_Motor/conversion 2/Over Ride6
  Over Ride7 : Soft_ECUs/softECU_Motor/conversion 2/Over Ride7
  Over Ride8 : Soft_ECUs/softECU_Motor/conversion 2/Over Ride8
  Over Ride9 : Soft_ECUs/softECU_Motor/conversion 2/Over Ride9
  Unit Delay : UnitDelay  SampleTime=-1
  Unit Delay1 : UnitDelay  SampleTime=-1
  MotorToHSC : Outport
  MotorTrqCMD : Outport  Port=2
  wires:
  Data Type Conversion13/1 -> Over Ride13/1
  Over Ride10/1 -> Bus Creator/11  "mot_REGID"
  StatusRequest/1 -> Data Type Conversion10/1
  MotorState/1 -> Data Type Conversion19/1
  Over Ride8/1 -> Bus Creator/9  "mot_run"
  Constant10/1 -> Data Type Conversion30/1
  Bus Selector1/3 -> Data Type Conversion3/1  "<MotPwrElec>"
  Over Ride9/1 -> Bus Creator/10  "mot_btb"
  Data Type Conversion9/1 -> Over Ride9/1
  Data Type Conversion21/1 -> Over Ride21/1
  StartupSignals/1 -> Bus Selector4/1
  MotorSignals/1 -> Bus Selector1/1
  Bus Selector4/2 -> Data Type Conversion9/1  "<mot_btb>"
  Bus Selector1/2 -> Data Type Conversion2/1  "<MotSpd>"
  Data Type Conversion5/1 -> Over Ride5/1
  Data Type Conversion28/1 -> Over Ride28/1
  Bus Selector4/1 -> Data Type Conversion8/1  "<mot_run>"
  Bus Selector1/7 -> Data Type Conversion7/1  "<mot_voltage>"
  Current_Override/1 -> Gain/1
  Bus Selector3/1 -> Data Type Conversion14/1  "<mot_fault_pwrVoltage>"
  Over Ride18/1 -> Bus Creator1/16  "mot_fault_iPeak"
  Over Ride16/1 -> Bus Creator1/14  "mot_fault_deviceTemp"
  Over Ride14/1 -> Bus Creator1/12  "mot_fault_pwrVoltage"
  Data Type Conversion1/1 -> Over Ride1/1
  Constant9/1 -> Data Type Conversion29/1
  Constant/1 -> Data Type Conversion20/1
  Data Type Conversion10/1 -> Over Ride10/1
  Data Type Conversion23/1 -> Over Ride23/1
  Data Type Conversion3/1 -> Over Ride3/1
  Data Type Conversion8/1 -> Over Ride8/1
  Data Type Conversion4/1 -> Over Ride4/1
  Bus Selector1/1 -> Data Type Conversion1/1  "<MotPwrMech>"
  Bus Selector1/5 -> Data Type Conversion5/1, Data Type Conversion11/1  "<mot temp>"
  Over Ride3/1 -> Bus Creator/4  "MOT_SerTx_getPwrEle"
  Over Ride5/1 -> Bus Creator/6  "mot_mtrTemp_degC"
  FaultDiagnos/1 -> Bus Selector3/1
  Bus Selector3/2 -> Data Type Conversion15/1  "<mot_fault_mtrTemp>"
  Bus Selector3/3 -> Data Type Conversion16/1  "<mot_fault_deviceTemp>"
  Data Type Conversion20/1 -> Over Ride20/1
  Constant11/1 -> Data Type Conversion13/1
  Data Type Conversion24/1 -> Over Ride24/1
  Over Ride7/1 -> Bus Creator/8  "mot_busVolt_V"
  Data Type Conversion19/1 -> Over Ride19/1
  Over Ride13/1 -> Bus Creator/13  "mot_positionAct"
  Over Ride19/1 -> Bus Creator/1  "mot_state"
  Bus Creator1/1 -> Fault insertion/1
  Data Type Conversion22/1 -> Over Ride22/1
  Gain2/1 -> Bus Creator/3  "mot_speedAct"
  Over Ride21/1 -> Bus Creator1/2  "mot_fault_pwr"
  Over Ride15/1 -> Bus Creator1/13  "mot_fault_mtrTemp"
  Data Type Conversion2/1 -> Over Ride2/1
  Data Type Conversion7/1 -> Over Ride7/1
  Over Ride20/1 -> Bus Creator1/1  "mot_fault_badParas"
  Data Type Conversion30/1 -> Over Ride30/1
  Bus Creator/1 -> MotorToHSC/1
  Over Ride6/1 -> Bus Creator/15  "mot_outTemp_degC"
  Over Ride25/1 -> Bus Creator1/6  "mot_fault_raceaway"
  Bus Selector3/4 -> Data Type Conversion17/1  "<mot_fault_overVoltage>"
  Over Ride1/1 -> Bus Creator/2  "MOT_SerTx_getPwrMech"
  Over Ride30/1 -> Bus Creator1/11  "mot_fault_ballast"
  Constant7/1 -> Data Type Conversion27/1
  Unit Delay/1 -> Bus Creator/12  "mot_currentSensor"
  Data Type Conversion18/1 -> Over Ride18/1
  Bus Selector1/8 -> Gain1/1  "<mot_currentSensor>"
  Gain1/1 -> Unit Delay/1
  Data Type Conversion11/1 -> Over Ride6/1
  Data Type Conversion12/1 -> Over Ride11/1
  Constant8/1 -> Data Type Conversion28/1
  Data Type Conversion6/1 -> Current_Override/1
  Data Type Conversion16/1 -> Over Ride16/1
  Over Ride22/1 -> Bus Creator1/3  "mot_fault_rfe"
  Constant1/1 -> Data Type Conversion21/1
  Data Type Conversion29/1 -> Over Ride29/1
  Fault insertion/1 -> Bus Creator/14  "mot_fault"
  Constant3/1 -> Data Type Conversion23/1
  Over Ride26/1 -> Bus Creator1/7  "mot_fault_canInit"
  Over Ride4/1 -> Bus Creator/5  "MOT_SerTx_getEff_k"
  Constant2/1 -> Data Type Conversion22/1
  Data Type Conversion14/1 -> Over Ride14/1
  Bus Selector1/4 -> Data Type Conversion4/1  "<MotEff_k>"
  Over Ride11/1 -> Bus Creator/16  "mot_inTemp_degC"
  Data Type Conversion25/1 -> Over Ride25/1
  Constant5/1 -> Data Type Conversion25/1
  Bus Selector1/6 -> Data Type Conversion6/1  "<mot_current>"
  Data Type Conversion26/1 -> Over Ride26/1
  Data Type Conversion27/1 -> Over Ride27/1
  Over Ride24/1 -> Bus Creator1/5  "mot_fault_resolver"
  Gain/1 -> Unit Delay1/1
  Over Ride2/1 -> Gain2/1  "mot_speedAct"
  Unit Delay1/1 -> Bus Creator/7  "mot_currentAct"
  Bus Selector3/5 -> Data Type Conversion18/1  "<mot_fault_iPeak>"
  Over Ride28/1 -> Bus Creator1/9  "mot_fault_encoder"
  Data Type Conversion17/1 -> Over Ride17/1
  Constant12/1 -> Data Type Conversion12/1
  Over Ride27/1 -> Bus Creator1/8  "mot_fault_adcInit"
  Over Ride17/1 -> Bus Creator1/15  "mot_fault_overVoltage"
  Over Ride23/1 -> Bus Creator1/4  "mot_fault_busTimeout"
  Data Type Conversion15/1 -> Over Ride15/1
  Constant6/1 -> Data Type Conversion26/1
  Constant4/1 -> Data Type Conversion24/1
  Over Ride29/1 -> Bus Creator1/10  "mot_fault_softError"
  MotorCMD/1 -> MotorTrqCMD/1

== system fullVehicleModel_17b/Vehicle Model/Variant Subsystem/Subsystem/Battery Thermal/Batt_overtemp_fault ==
  note: Override Switch Subsystem
  note: This subsystem is used to override the model value of a signal to a constant value
  Power : Inport
  Temp : Inport  Port=2
  First Degree Fault : Subsystem
  Multiport Switch : MultiPortSwitch  DataPortOrder=Zero-based contiguous  zeroidx=on
  Second Degree Fault : Subsystem
  override_flag : Constant  Value=0
  Out1 : Outport
  wires:
  First Degree Fault/1(Out1) -> Multiport Switch/3
  Second Degree Fault/1(Out1) -> Multiport Switch/4
  Power/1 -> First Degree Fault/3(Power)
  Multiport Switch/1 -> Out1/1, Second Degree Fault/1(In1)
  override_flag/1 -> Multiport Switch/1, First Degree Fault/1(Flag)
  Temp/1 -> First Degree Fault/2(Temp), Multiport Switch/2

== system fullVehicleModel_17b/Vehicle Model/Variant Subsystem/Subsystem/Battery Thermal/M1 to Scope ==
  PS-Simulink Converter : nesl_utility/PS-Simulink Converter  PhysicalDomain=network_engine_domain  SubClassName=ps_output  LeftPortType=input  RightPortType=output  PseudoPeriodic=off  Frequencies=[]  Unit=1  AffineConversion=off
  Rate Transition : RateTransition
  Temperature Conversion : aerolibconvert2/Temperature Conversion  IU=K  OU=C
      settings: SourceProductName=Aerospace Blockset  SourceProductBaseCode=AE
  Conn1 : PMIOPort  Port=1  Side=Left
  Out1 : Outport
  wires:
  Rate Transition/1 -> Temperature Conversion/1
  PS-Simulink Converter/1 -> Rate Transition/1
  Temperature Conversion/1 -> Out1/1
  connections:
  PS-Simulink Converter/LConn1 -- Conn1/RConn1

== system fullVehicleModel_17b/Vehicle Model/Variant Subsystem/Subsystem/Battery Thermal/M2 to scope ==
  PS-Simulink Converter : nesl_utility/PS-Simulink Converter  PhysicalDomain=network_engine_domain  SubClassName=ps_output  LeftPortType=input  RightPortType=output  PseudoPeriodic=off  Frequencies=[]  Unit=1  AffineConversion=off
  Rate Transition : RateTransition
  Temperature Conversion : aerolibconvert2/Temperature Conversion  IU=K  OU=C
      settings: SourceProductName=Aerospace Blockset  SourceProductBaseCode=AE
  Conn1 : PMIOPort  Port=1  Side=Left
  Out1 : Outport
  wires:
  Rate Transition/1 -> Temperature Conversion/1
  Temperature Conversion/1 -> Out1/1
  PS-Simulink Converter/1 -> Rate Transition/1
  connections:
  PS-Simulink Converter/LConn1 -- Conn1/RConn1

== system fullVehicleModel_17b/Vehicle Model/Variant Subsystem/Subsystem/Battery Thermal/M3 to scope ==
  PS-Simulink Converter : nesl_utility/PS-Simulink Converter  PhysicalDomain=network_engine_domain  SubClassName=ps_output  LeftPortType=input  RightPortType=output  PseudoPeriodic=off  Frequencies=[]  Unit=1  AffineConversion=off
  Rate Transition : RateTransition
  Temperature Conversion : aerolibconvert2/Temperature Conversion  IU=K  OU=C
      settings: SourceProductName=Aerospace Blockset  SourceProductBaseCode=AE
  Conn1 : PMIOPort  Port=1  Side=Left
  Out1 : Outport
  wires:
  Rate Transition/1 -> Temperature Conversion/1
  Temperature Conversion/1 -> Out1/1
  PS-Simulink Converter/1 -> Rate Transition/1
  connections:
  PS-Simulink Converter/LConn1 -- Conn1/RConn1

== system fullVehicleModel_17b/Vehicle Model/Variant Subsystem/Subsystem/Battery Thermal/M4 to scope ==
  PS-Simulink Converter : nesl_utility/PS-Simulink Converter  PhysicalDomain=network_engine_domain  SubClassName=ps_output  LeftPortType=input  RightPortType=output  PseudoPeriodic=off  Frequencies=[]  Unit=1  AffineConversion=off
  Rate Transition : RateTransition
  Temperature Conversion : aerolibconvert2/Temperature Conversion  IU=K  OU=C
      settings: SourceProductName=Aerospace Blockset  SourceProductBaseCode=AE
  Conn1 : PMIOPort  Port=1  Side=Left
  Out1 : Outport
  wires:
  Rate Transition/1 -> Temperature Conversion/1
  Temperature Conversion/1 -> Out1/1
  PS-Simulink Converter/1 -> Rate Transition/1
  connections:
  PS-Simulink Converter/LConn1 -- Conn1/RConn1

== system fullVehicleModel_17b/Vehicle Model/Variant Subsystem/Subsystem/Battery Thermal/M5 to scope ==
  PS-Simulink Converter : nesl_utility/PS-Simulink Converter  PhysicalDomain=network_engine_domain  SubClassName=ps_output  LeftPortType=input  RightPortType=output  PseudoPeriodic=off  Frequencies=[]  Unit=1  AffineConversion=off
  Rate Transition : RateTransition
  Temperature Conversion : aerolibconvert2/Temperature Conversion  IU=K  OU=C
      settings: SourceProductName=Aerospace Blockset  SourceProductBaseCode=AE
  Conn1 : PMIOPort  Port=1  Side=Left
  Out1 : Outport
  wires:
  Rate Transition/1 -> Temperature Conversion/1
  Temperature Conversion/1 -> Out1/1
  PS-Simulink Converter/1 -> Rate Transition/1
  connections:
  PS-Simulink Converter/LConn1 -- Conn1/RConn1

== system fullVehicleModel_17b/Vehicle Model/Variant Subsystem/Subsystem/Battery Thermal/M6 to Scope ==
  PS-Simulink Converter : nesl_utility/PS-Simulink Converter  PhysicalDomain=network_engine_domain  SubClassName=ps_output  LeftPortType=input  RightPortType=output  PseudoPeriodic=off  Frequencies=[]  Unit=1  AffineConversion=off
  Rate Transition : RateTransition
  Temperature Conversion : aerolibconvert2/Temperature Conversion  IU=K  OU=C
      settings: SourceProductName=Aerospace Blockset  SourceProductBaseCode=AE
  Conn1 : PMIOPort  Port=1  Side=Left
  Out1 : Outport
  wires:
  Rate Transition/1 -> Temperature Conversion/1
  PS-Simulink Converter/1 -> Rate Transition/1
  Temperature Conversion/1 -> Out1/1
  connections:
  PS-Simulink Converter/LConn1 -- Conn1/RConn1

== system fullVehicleModel_17b/Vehicle Model/Variant Subsystem/Subsystem/Battery Thermal/M7 to scope ==
  PS-Simulink Converter : nesl_utility/PS-Simulink Converter  PhysicalDomain=network_engine_domain  SubClassName=ps_output  LeftPortType=input  RightPortType=output  PseudoPeriodic=off  Frequencies=[]  Unit=1  AffineConversion=off
  Rate Transition : RateTransition
  Temperature Conversion : aerolibconvert2/Temperature Conversion  IU=K  OU=C
      settings: SourceProductName=Aerospace Blockset  SourceProductBaseCode=AE
  Conn1 : PMIOPort  Port=1  Side=Left
  Out1 : Outport
  wires:
  Rate Transition/1 -> Temperature Conversion/1
  PS-Simulink Converter/1 -> Rate Transition/1
  Temperature Conversion/1 -> Out1/1
  connections:
  PS-Simulink Converter/LConn1 -- Conn1/RConn1

== system fullVehicleModel_17b/Vehicle Model/Variant Subsystem/Subsystem/Battery Thermal/Module 1 ==
  Power Cycle : Inport
  Ideal Heat Flow Source : fl_lib/Thermal/Thermal Sources/Controlled Heat Flow Rate Source
      settings: SourceProductName=Simscape
  Ideal Temperature Sensor : fl_lib/Thermal/Thermal Sensors/Temperature Sensor
  Simulink-PS Converter1 : nesl_utility/Simulink-PS Converter  PhysicalDomain=network_engine_domain  SubClassName=ps_input  LeftPortType=input  RightPortType=output  PseudoPeriodic=off  Frequencies=[]  NoiseDistribution=none  NoiseParameters=[]  Unit=1  AffineConversion=off  FilteringAndDerivatives=zero  SimscapeFilterOrder=1  InputFilterTimeConstant=0.001  UdotUserProvided=1
  Thermal Mass : fl_lib/Thermal/Thermal Elements/Thermal Mass  mass=module_mass kg  sp_heat=specific_heat_module J/kg/K  T_specify=on  T_priority=High  T=ambient_temp K  T_nominal_specify=off  T_nominal_unit=K  T_nominal_value=1  Q_specify=off  Q_priority=High  Q=0 J/s  Q_nominal_specify=off  Q_nominal_unit=W  Q_nominal_value=1
  Thermal Reference1 : fl_lib/Thermal/Thermal Elements/Thermal Reference
  Thermal Reference2 : fl_lib/Thermal/Thermal Elements/Thermal Reference
  Temperature : PMIOPort  Port=1  Side=Right
  Air Convection : PMIOPort  Port=2  Side=Right
  Convection from Module 6 : PMIOPort  Port=3  Side=Left
  Convection from Module 2 : PMIOPort  Port=4  Side=Left
  wires:
  Power Cycle/1 -> Simulink-PS Converter1/1
  connections:
  Ideal Heat Flow Source/RConn1 -- Simulink-PS Converter1/RConn1
  Thermal Reference2/LConn1 -- Ideal Heat Flow Source/RConn2
  Temperature/RConn1 -- Ideal Temperature Sensor/RConn2
  Thermal Reference1/LConn1 -- Ideal Temperature Sensor/RConn1
  Convection from Module 2/RConn1 -- Convection from Module 6/RConn1 -- Ideal Heat Flow Source/LConn1 -- Ideal Temperature Sensor/LConn1 -- Thermal Mass/LConn1 -- Air Convection/RConn1

== system fullVehicleModel_17b/Vehicle Model/Variant Subsystem/Subsystem/Battery Thermal/Module 2 ==
  Power Cycle : Inport
  Ideal Heat Flow Source : fl_lib/Thermal/Thermal Sources/Controlled Heat Flow Rate Source
      settings: SourceProductName=Simscape
  Ideal Temperature Sensor : fl_lib/Thermal/Thermal Sensors/Temperature Sensor
  Simulink-PS Converter1 : nesl_utility/Simulink-PS Converter  PhysicalDomain=network_engine_domain  SubClassName=ps_input  LeftPortType=input  RightPortType=output  PseudoPeriodic=off  Frequencies=[]  NoiseDistribution=none  NoiseParameters=[]  Unit=1  AffineConversion=off  FilteringAndDerivatives=zero  SimscapeFilterOrder=1  InputFilterTimeConstant=0.001  UdotUserProvided=1
  Thermal Mass : fl_lib/Thermal/Thermal Elements/Thermal Mass  mass=module_mass kg  sp_heat=specific_heat_module J/kg/K  T_specify=on  T_priority=High  T=ambient_temp K  T_nominal_specify=off  T_nominal_unit=K  T_nominal_value=1  Q_specify=off  Q_priority=High  Q=0 J/s  Q_nominal_specify=off  Q_nominal_unit=W  Q_nominal_value=1
  Thermal Reference1 : fl_lib/Thermal/Thermal Elements/Thermal Reference
  Thermal Reference2 : fl_lib/Thermal/Thermal Elements/Thermal Reference
  Temperature : PMIOPort  Port=1  Side=Right
  Air Convection : PMIOPort  Port=2  Side=Right
  Convection from Module 1 : PMIOPort  Port=3  Side=Left
  wires:
  Power Cycle/1 -> Simulink-PS Converter1/1
  connections:
  Ideal Heat Flow Source/RConn1 -- Simulink-PS Converter1/RConn1
  Thermal Reference2/LConn1 -- Ideal Heat Flow Source/RConn2
  Temperature/RConn1 -- Ideal Temperature Sensor/RConn2
  Thermal Reference1/LConn1 -- Ideal Temperature Sensor/RConn1
  Ideal Heat Flow Source/LConn1 -- Convection from Module 1/RConn1 -- Ideal Temperature Sensor/LConn1 -- Thermal Mass/LConn1 -- Air Convection/RConn1

== system fullVehicleModel_17b/Vehicle Model/Variant Subsystem/Subsystem/Battery Thermal/Module 3 ==
  Power Cycle : Inport
  Ideal Heat Flow Source : fl_lib/Thermal/Thermal Sources/Controlled Heat Flow Rate Source
      settings: SourceProductName=Simscape
  Ideal Temperature Sensor : fl_lib/Thermal/Thermal Sensors/Temperature Sensor
  Simulink-PS Converter1 : nesl_utility/Simulink-PS Converter  PhysicalDomain=network_engine_domain  SubClassName=ps_input  LeftPortType=input  RightPortType=output  PseudoPeriodic=off  Frequencies=[]  NoiseDistribution=none  NoiseParameters=[]  Unit=1  AffineConversion=off  FilteringAndDerivatives=zero  SimscapeFilterOrder=1  InputFilterTimeConstant=0.001  UdotUserProvided=1
  Thermal Mass : fl_lib/Thermal/Thermal Elements/Thermal Mass  mass=module_mass kg  sp_heat=specific_heat_module J/kg/K  T_specify=on  T_priority=High  T=ambient_temp K  T_nominal_specify=off  T_nominal_unit=K  T_nominal_value=1  Q_specify=off  Q_priority=High  Q=0 J/s  Q_nominal_specify=off  Q_nominal_unit=W  Q_nominal_value=1
  Thermal Reference1 : fl_lib/Thermal/Thermal Elements/Thermal Reference
  Thermal Reference2 : fl_lib/Thermal/Thermal Elements/Thermal Reference
  Temperature : PMIOPort  Port=1  Side=Right
  Air Convection : PMIOPort  Port=2  Side=Right
  Convection from Module 4 : PMIOPort  Port=3  Side=Left
  Convection from Electronics : PMIOPort  Port=4  Side=Left
  wires:
  Power Cycle/1 -> Simulink-PS Converter1/1
  connections:
  Simulink-PS Converter1/RConn1 -- Ideal Heat Flow Source/RConn1
  Thermal Reference2/LConn1 -- Ideal Heat Flow Source/RConn2
  Temperature/RConn1 -- Ideal Temperature Sensor/RConn2
  Thermal Reference1/LConn1 -- Ideal Temperature Sensor/RConn1
  Ideal Heat Flow Source/LConn1 -- Convection from Module 4/RConn1 -- Convection from Electronics/RConn1 -- Ideal Temperature Sensor/LConn1 -- Thermal Mass/LConn1 -- Air Convection/RConn1

== system fullVehicleModel_17b/Vehicle Model/Variant Subsystem/Subsystem/Battery Thermal/Module 4 ==
  Power Cycle : Inport
  Ideal Temperature Sensor : fl_lib/Thermal/Thermal Sensors/Temperature Sensor
  Simulink-PS Converter1 : nesl_utility/Simulink-PS Converter  PhysicalDomain=network_engine_domain  SubClassName=ps_input  LeftPortType=input  RightPortType=output  PseudoPeriodic=off  Frequencies=[]  NoiseDistribution=none  NoiseParameters=[]  Unit=1  AffineConversion=off  FilteringAndDerivatives=zero  SimscapeFilterOrder=1  InputFilterTimeConstant=0.001  UdotUserProvided=1
  Thermal Energy of Cells : fl_lib/Thermal/Thermal Sources/Controlled Heat Flow Rate Source
      settings: SourceProductName=Simscape
  Thermal Mass : fl_lib/Thermal/Thermal Elements/Thermal Mass  mass=module_mass kg  sp_heat=specific_heat_module J/kg/K  T_specify=on  T_priority=High  T=ambient_temp K  T_nominal_specify=off  T_nominal_unit=K  T_nominal_value=1  Q_specify=off  Q_priority=High  Q=0 J/s  Q_nominal_specify=off  Q_nominal_unit=W  Q_nominal_value=1
  Thermal Reference1 : fl_lib/Thermal/Thermal Elements/Thermal Reference
  Thermal Reference2 : fl_lib/Thermal/Thermal Elements/Thermal Reference
  Temperature : PMIOPort  Port=1  Side=Right
  Air Convection : PMIOPort  Port=2  Side=Right
  Convection from Module 3 : PMIOPort  Port=3  Side=Left
  Convection from Module 5 : PMIOPort  Port=4  Side=Left
  Convection from Electronics : PMIOPort  Port=5  Side=Left
  wires:
  Power Cycle/1 -> Simulink-PS Converter1/1
  connections:
  Thermal Energy of Cells/RConn1 -- Simulink-PS Converter1/RConn1
  Thermal Reference2/LConn1 -- Thermal Energy of Cells/RConn2
  Temperature/RConn1 -- Ideal Temperature Sensor/RConn2
  Thermal Reference1/LConn1 -- Ideal Temperature Sensor/RConn1
  Thermal Energy of Cells/LConn1 -- Convection from Module 5/RConn1 -- Convection from Module 3/RConn1 -- Convection from Electronics/RConn1 -- Ideal Temperature Sensor/LConn1 -- Thermal Mass/LConn1 -- Air Convection/RConn1
